simulink model "Joystick"  (R2021b)
settings: Solver=FixedStepAuto  StartTime=0.0  StopTime=inf  RelTol=1e-3
libraries: arduinolib x13
settings Model: ExtModeTrigDuration=2  Creator=maqui  LastModifiedBy=maqui
settings OptimizationCC: EnhancedBackFolding=on  PassReuseOutputArgsAs=Individual arguments  ZeroExternalMemoryAtStartup=off  ZeroInternalMemoryAtStartup=off  MaxStackSize=64  OptimizeBlockOrder=speed  DifferentSizesBufferReuse=on  OptimizationCustomize=off  EfficientTunableParamExpr=on
settings DebuggingCC: ParameterTunabilityLossMsg=error
settings HardwareCC: ProdBitPerInt=16  ProdBitPerPointer=16  ProdBitPerSizeT=16  ProdBitPerPtrDiffT=16  ProdLargestAtomicFloat=None  ProdWordSize=8  ProdHWDeviceType=Atmel->AVR  UseEmbeddedCoderFeatures=off  UseSimulinkCoderFeatures=off
settings SFSimCC: MATLABDynamicMemAlloc=off
settings RTWCC: Description=Embedded Coder  SystemTargetFile=ert.tlc  HardwareBoard=Arduino Uno  TemplateMakefile=ert_default_tmf  Toolchain=Arduino AVR
settings CodeAppCC: ForceParamTrailComments=on  IgnoreCustomStorageClasses=off  OperatorAnnotations=on  SimulinkDataObjDesc=on  SFDataObjDesc=on  InsertBlockDesc=on
settings ERTTargetCC: SupportContinuousTime=on  SupportNonInlinedSFcns=on  SupportVariableSizeSignals=on  ExtModeTransport=3  ExtModeStaticAlloc=on  ExtModeStaticAllocSize=250  ExtModeMexFile=ext_xcp  ExtModeIntrfLevel=Level2 - Open

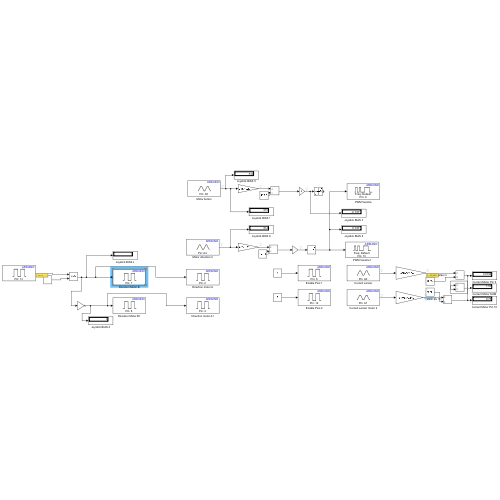
[thumbnail: Simulink's stored preview of the top-level diagram]
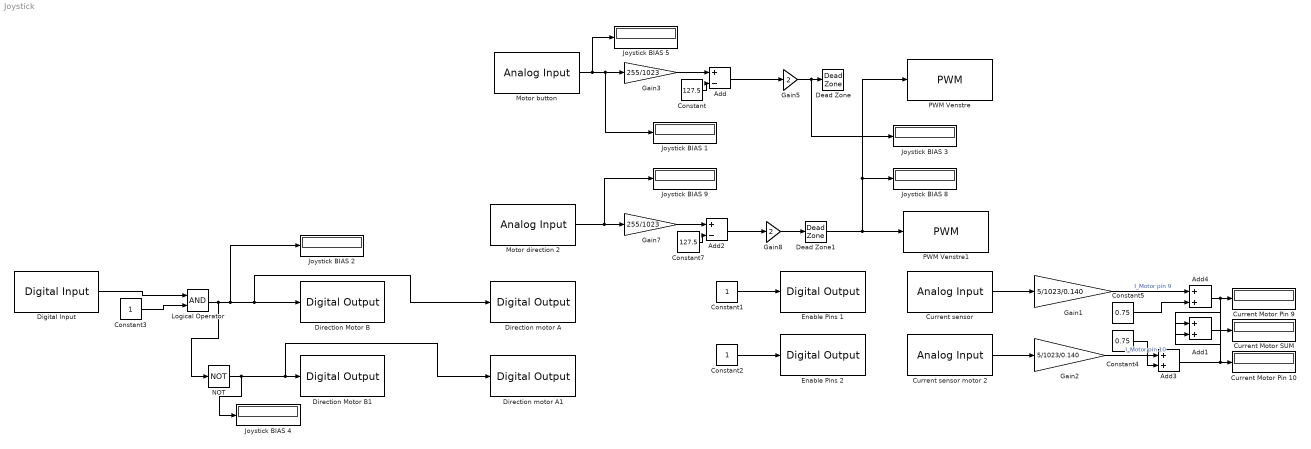
== system Joystick ==
  Add : Sum  Inputs=+-
  Add1 : Sum
  Add2 : Sum  Inputs=+-
  Add3 : Sum
  Add4 : Sum
  Constant : Constant  Value=127.5
  Constant1 : Constant
  Constant2 : Constant
  Constant3 : Constant
  Constant4 : Constant  Value=0.75
  Constant5 : Constant  Value=0.75
  Constant7 : Constant  Value=127.5
  Current Motor Pin 10 : Display
  Current Motor Pin 9 : Display
  Current Motor SUM : Display
  Current sensor : arduinolib/Analog Input  pinNumber=0  ReadResultsOnly=off  ConversionTriggerSource=Software  ExternalTriggerType=uint32( 0 )  OutputDataType=uint16  EnableConversionCompleteNotify=off  EnableOuputStatus=off  SampleTime=-1  blockPlatform=arduino
  Current sensor motor 2 : arduinolib/Analog Input  pinNumber=1  ReadResultsOnly=off  ConversionTriggerSource=Software  ExternalTriggerType=uint32( 0 )  OutputDataType=uint16  EnableConversionCompleteNotify=off  EnableOuputStatus=off  SampleTime=-1  blockPlatform=arduino
  Dead Zone : DeadZone  SaturateOnIntegerOverflow=on
  Dead Zone1 : DeadZone  SaturateOnIntegerOverflow=on
  Digital Input : arduinolib/Digital Input  pinNumber=13  mode=Input Pullup  Direction=input  SampleTime=-1  blockPlatform=arduino
  Direction Motor B : arduinolib/Digital Output  pinNumber=7  Direction=output  blockPlatform=arduino
  Direction Motor B1 : arduinolib/Digital Output  pinNumber=8  Direction=output  blockPlatform=arduino
  Direction motor A : arduinolib/Digital Output  pinNumber=2  Direction=output  blockPlatform=arduino
  Direction motor A1 : arduinolib/Digital Output  pinNumber=4  Direction=output  blockPlatform=arduino
  Enable Pins 1 : arduinolib/Digital Output  pinNumber=6  Direction=output  blockPlatform=arduino
  Enable Pins 2 : arduinolib/Digital Output  pinNumber=12  Direction=output  blockPlatform=arduino
  Gain1 : Gain  Gain=5/1023/0.140
  Gain2 : Gain  Gain=5/1023/0.140
  Gain3 : Gain  Gain=255/1023
  Gain5 : Gain  Gain=2
  Gain7 : Gain  Gain=255/1023
  Gain8 : Gain  Gain=2
  Joystick BIAS {1..5,8..9} (7 alike) : Display
  Logical Operator : Logic  AllPortsSameDT=off  OutDataTypeStr=boolean
  Motor button : arduinolib/Analog Input  pinNumber=5  ReadResultsOnly=off  ConversionTriggerSource=Software  ExternalTriggerType=uint32( 0 )  OutputDataType=uint16  EnableConversionCompleteNotify=off  EnableOuputStatus=off  SampleTime=-1  blockPlatform=arduino
  Motor direction 2 : arduinolib/Analog Input  pinNumber=4  ReadResultsOnly=off  ConversionTriggerSource=Software  ExternalTriggerType=uint32( 0 )  OutputDataType=uint16  EnableConversionCompleteNotify=off  EnableOuputStatus=off  SampleTime=-1  blockPlatform=arduino
  NOT : Logic  Operator=NOT  IconShape=distinctive  AllPortsSameDT=off  OutDataTypeStr=boolean
  PWM Venstre : arduinolib/PWM  pinNumber=9  frequencyType=Default  desiredFrequency=490.2  achievableFrequency=490.2
  PWM Venstre1 : arduinolib/PWM  pinNumber=10  frequencyType=Default  desiredFrequency=490.2  achievableFrequency=490.2
  wires:
  Constant1/1 -> Enable Pins 1/1
  Constant2/1 -> Enable Pins 2/1
  Current sensor/1 -> Gain1/1
  Motor button/1 -> Joystick BIAS 5/1, Joystick BIAS 1/1, Gain3/1
  Constant/1 -> Add/2
  Add/1 -> Gain5/1
  Current sensor motor 2/1 -> Gain2/1
  Gain3/1 -> Add/1
  Gain5/1 -> Joystick BIAS 3/1, Dead Zone/1
  Gain7/1 -> Add2/1
  Add2/1 -> Gain8/1
  Motor direction 2/1 -> Joystick BIAS 9/1, Gain7/1
  Constant7/1 -> Add2/2
  NOT/1 -> Joystick BIAS 4/1, Direction motor A1/1, Direction Motor B1/1
  Logical Operator/1 -> NOT/1, Direction motor A/1, Direction Motor B/1, Joystick BIAS 2/1
  Constant3/1 -> Logical Operator/2
  Digital Input/1 -> Logical Operator/1
  Add1/1 -> Current Motor SUM/1
  Constant4/1 -> Add3/2
  Gain2/1 -> Add3/1  "I_Motor pin 10"
  Add3/1 -> Add1/2, Current Motor Pin 10/1
  Add4/1 -> Add1/1, Current Motor Pin 9/1
  Constant5/1 -> Add4/2
  Gain1/1 -> Add4/1  "I_Motor pin 9"
  Gain8/1 -> Dead Zone1/1
  Dead Zone1/1 -> Joystick BIAS 8/1, PWM Venstre/1, PWM Venstre1/1
